simulink model "simplified"  (Simulink 8.6)
settings: Solver=FixedStepAuto  SolverMode=SingleTasking  StartTime=0.0  StopTime=300  FixedStep=1e-3  RelTol=1e-3
libraries: simulink x7
settings Model: Creator=z003vh9b  LastModifiedBy=z003vh9b
settings DataIOCC: LimitDataPoints=off  SaveFormat=Dataset  SignalLoggingSaveFormat=Dataset
settings OptimizationCC: ExpressionDepthLimit=128
settings DebuggingCC: UnderspecifiedInitializationDetection=Simplified  MergeDetectMultiDrivingBlocksExec=error  SolverPrmCheckMsg=none  FcnCallInpInsideContextMsg=EnableAllAsError  AllowSymbolicDim=on  StateNameClashWarn=none  SFUnexpectedBacktrackingDiag=error  SFNoUnconditionalDefaultTransitionDiag=error
settings HardwareCC: ProdBitPerPointer=64  ProdLargestAtomicFloat=Float  ProdIntDivRoundTo=Zero  ProdEndianess=LittleEndian  ProdWordSize=64  ProdHWDeviceType=Intel->x86-64 (Windows64)
settings ModelReferenceCC: PropagateSignalLabelsOutOfModel=on
settings GRTTargetCC: TargetLangStandard=C99 (ISO)  GeneratePreprocessorConditionals=Use local settings  CombineOutputUpdateFcns=on  GRTInterface=off
settings ConfigComp: CovMetricSettings=dwe  CovHtmlReporting=off  CovSaveCumulativeToWorkspaceVar=off  CovSaveSingleToWorkspaceVar=off  CovExternalEMLEnable=on

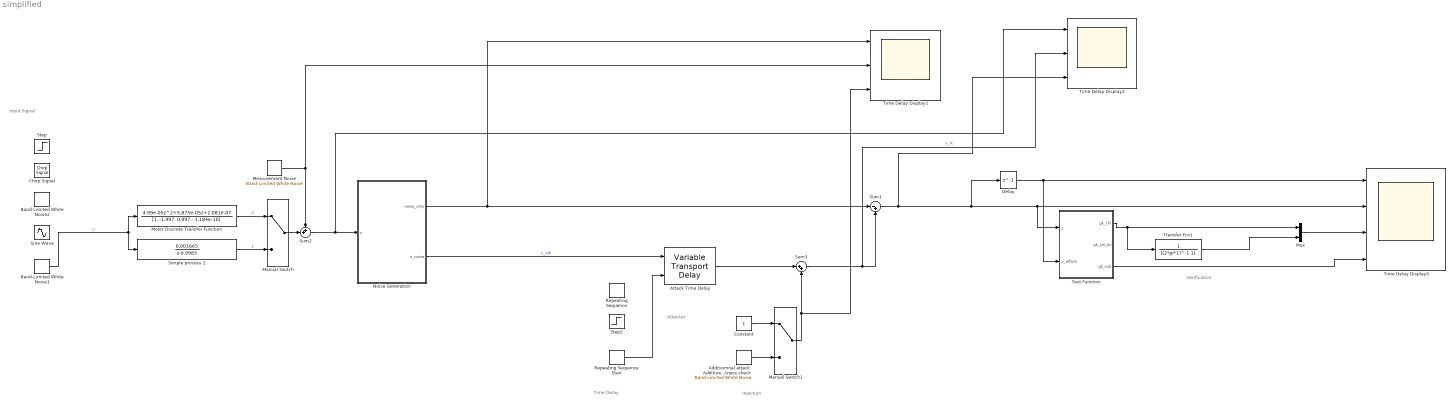
== system simplified ==
  note: Input Signal
  note: Time Delay
  note: Attacker
  note: Injection
  note: Verificaiton
  "Additiomnal attack  Additive Noise  Robustness check " : simulink/Sources/Band-Limited White Noise  Cov=[1e-8]  Ts=1e-3  seed=[233241]
  Attack Time Delay : VariableTransportDelay  MaximumDelay=100  InitialOutput=2e-3  ZeroDelay=on
  Band-Limited White Noise1 : simulink/Sources/Band-Limited White Noise  Cov=[1e-3]  Ts=1  seed=[23324]
  Band-Limited White Noise2 : simulink/Sources/Band-Limited White Noise  Cov=[1e-3]  Ts=1e-2  seed=[23324]
  Chirp Signal : simulink/Sources/Chirp Signal  f1=0.1  T=300  f2=20*pi
  Constant : Constant
  Delay : Delay  DelayLength=1  InitialCondition=0
  Manual Switch : ManualSwitch
  Manual Switch1 : ManualSwitch
  Measurement Noise : simulink/Sources/Band-Limited White Noise  Cov=[1e-9]  Ts=1e-3  seed=[23341]
  Motor Discrete Transfer Function : DiscreteTransferFcn  Numerator=[4.99e-05, 5.875e-05, 2.081e-07]  Denominator=[1, -1.997, 0.997,- 1.184e-10]  SampleTime=1e-3
  Mux : Mux  Inputs=2
  Noise Generation : MATLAB Function  TreatAsAtomicUnit=on
      settings: PermitHierarchicalResolution=ParametersOnly
  Repeating Sequence : simulink/Sources/Repeating Sequence  rep_seq_t=[1:5:100]  rep_seq_y=[1:1:20]*1e-3
  Repeating Sequence Stair : simulink/Sources/Repeating Sequence Stair  OutValues=[2e-3 0e-3 15e-3 4e-3 0e-3 8e-3].'  tsamp=40  OutMin=[]  OutMax=[]  OutDataTypeStr=double  OutputDataTypeScalingMode=double  OutDataType=fixdt(0,8)  ConRadixGroup=Best Precision: Vector-wise  OutScaling=2^-12
  Simple process 1 : DiscreteTransferFcn  Numerator=[0.001665]  Denominator=[1, -0.9983]  SampleTime=1e-3
  Sine Wave : Sin  Frequency=0.1*pi  SampleTime=0
  Step : Step  Time=3  SampleTime=0
  Step2 : Step  Time=10  After=5e-3  SampleTime=0
  Sum1 : Sum  Inputs=|-+
  Sum2 : Sum  Inputs=++|
  Sum3 : Sum  Inputs=|++
  Test Function : MATLAB Function  TreatAsAtomicUnit=on  SystemSampleTime=1e-3
      settings: PermitHierarchicalResolution=ParametersOnly
  Time Delay Display1 : Scope  NumInputPorts=3
  Time Delay Display2 : Scope  NumInputPorts=3
  Time Delay Display5 : Scope  NumInputPorts=4
  Transfer Fcn1 : TransferFcn  Denominator=[(2*pi*1)^-1 1]
  wires:
  Simple process 1/1 -> Manual Switch/2  "y"
  Repeating Sequence Stair/1 -> Attack Time Delay/2
  Sum3/1 -> Time Delay Display2/2, Sum1/2  "y_rt"
  Measurement Noise/1 -> Sum2/1, Time Delay Display1/2
  Band-Limited White Noise1/1 -> Simple process 1/1, Motor Discrete Transfer Function/1  "u"
  Noise Generation/2(x_noise) -> Attack Time Delay/1  "y_eth"
  Attack Time Delay/1 -> Sum3/1
  Motor Discrete Transfer Function/1 -> Manual Switch/1  "y"
  Sum2/1 -> Time Delay Display2/1, Noise Generation/1(x)
  Noise Generation/1(noise_only) -> Time Delay Display1/1, Sum1/1
  Sum1/1 -> Time Delay Display2/3, Time Delay Display5/2, Test Function/1(y), Delay/1
  Delay/1 -> Test Function/2(y_attack), Time Delay Display5/1
  Test Function/1(gk_chi) -> Transfer Fcn1/1, Mux/1
  Transfer Fcn1/1 -> Mux/2
  Mux/1 -> Time Delay Display5/3
  Manual Switch1/1 -> Time Delay Display1/3, Sum3/2
  "Additiomnal attack  Additive Noise  Robustness check "/1 -> Manual Switch1/2
  Constant/1 -> Manual Switch1/1
  Test Function/3(gk_sub) -> Time Delay Display5/4
  Manual Switch/1 -> Sum2/2

== matlab function Noise Generation ==
  data: noise_only output double; x_noise output double; x input double
function [noise_only,   x_noise]= fcn(x)

Ts_IRT = 100e-6;
Ts_RT = 1e-3;
Ts = 100e-3;
Ts_SRT = 100e-3;
SensorCh = 1;
SensorNoise = 1;
NoiseMagnitude = 1e-3;

if ~SensorNoise 
    x_noise = x;
    noise_only = zeros(length(x),1);
    return;
end


persistent t noise ms register uniqueLength stages weights;
%% Initialisation
if isempty(t) 
    t=0;
    noise = zeros(length(x),1);
       
    % Random number algorithm intitialization 
%     stages = 5;
%     uniqueLength = 5;
%     weights=[1, 1, 2, 1, 2];

%     stages = 3;
%     uniqueLength = 5;
%     weights=[1,1,2,0,2];

%     stages = 3;
%     uniqueLength = 7;
%     weights=[0,2,2,1,2,2,2];

    stages = 7;
    uniqueLength = 5;
    weights=[1,3,1,4,3];

    
    register = round(rem(rand(length(x),uniqueLength)*stages,stages));

else
    t=t+1;
    
    if ~mod(t,Ts_SRT/Ts)
        % Re-inti value of the shiftReg every step of the Ethernet package
        % sent
    end
    
    % smart stuff RT
    if ~mod(t,Ts_RT/Ts) && SensorCh == 1
        
        ms=rem(register*weights'+stages,stages);
        register=[ms, register(:,1:uniqueLength-1)];
        noise = NoiseMagnitude'.* (ms - floor(stages/2)); % eg. 5 stages 0 1 2 3 4 5 -> -2 -1 0 1 2
    elseif  ~mod(t,Ts_IRT/Ts) && SensorCh == 2
        % smart stuff IRT


    end
end

noise_only = noise;
x_noise = x + noise;
end

function b = bipolar(a)
b = 2*a-1;
end

== matlab function Test Function ==
  data: y input double; gk_chi output double; gk_chi_av output double; y_attack input double; gk_sub output double
function [gk_chi,gk_chi_av, gk_sub] = fcn(y,y_attack)


persistent Y Y_attack Variance GK

wind =10;
if isempty(Y)
    Y = zeros(wind,1);
    Y_attack = zeros(wind,1);
    Variance = 1e-4;
    GK = zeros(wind,1);
else
    Y = [y; Y(1:end-1)];
    Y_attack = [y_attack; Y_attack(1:end-1)];
end

% mean = sum(Y_attack)/wind;
% stdev = 1/wind*sqrt(sum((Y_attack-wind).^2));
% gk = stdev;
gk_chi = sum((Y-Y_attack).*Variance^-1.*(Y-Y_attack));
gk_chi_av = abs(sum(GK))/wind;
GK = [gk_chi; GK(1:end-1)];
gk_sub = Y(1)-Y_attack(2);
